simulink model "sampleModel193"  (R2021b)
settings: Solver=VariableStepAuto  StartTime=0.0  StopTime=10.0  RelTol=1e-3
undefined symbols (not defined in the file or in its folder): Newton, Raphson
libraries: simulink x7, slpidlib x2
settings Model: Creator=user  LastModifiedBy=user

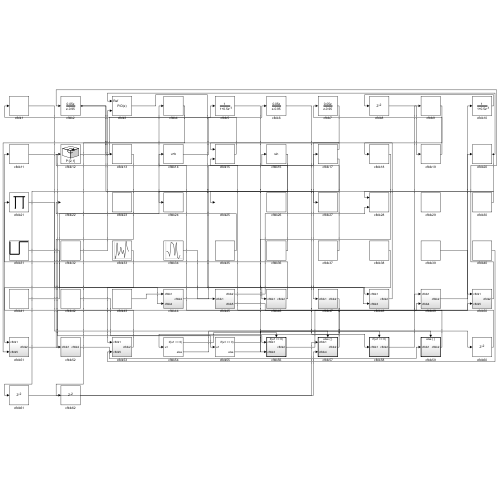
[thumbnail: Simulink's stored preview of the top-level diagram]
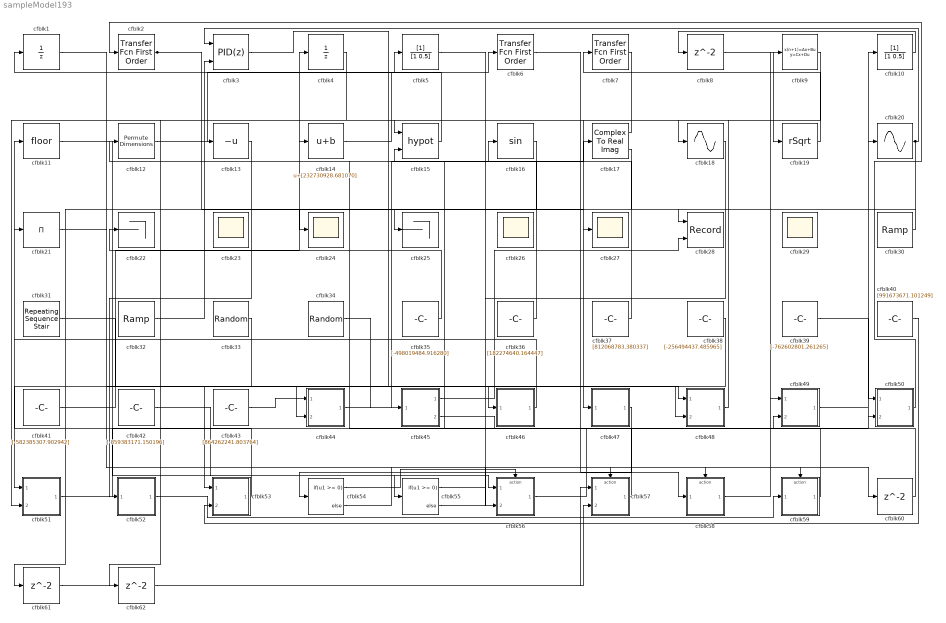
== system sampleModel193 ==
  cfblk1 : UnitDelay  HasFrameUpgradeWarning=on
  cfblk10 : DiscreteFilter  SampleTime=1
  cfblk11 : Rounding
  cfblk12 : PermuteDimensions
  cfblk13 : UnaryMinus
  cfblk14 : Bias  Bias=[232730928.681070]
  cfblk15 : Math  Operator=hypot  SaturateOnIntegerOverflow=on
  cfblk16 : Trigonometry
  cfblk17 : ComplexToRealImag
  cfblk18 : Sin  TimeSource=Use external signal  SampleTime=0
  cfblk19 : Sqrt  Operator=rSqrt  AlgorithmType=Newton-Raphson  SaturateOnIntegerOverflow=on
  cfblk2 : simulink/Discrete/Transfer Fcn First Order  PoleZ=0.95  ICPrevOutput=0.0  DoSatur=off
  cfblk20 : Sin  TimeSource=Use external signal  SampleTime=0
  cfblk21 : Product  Inputs=*
  cfblk22 : Terminator
  cfblk{23..24,26..27,29} (5 alike) : Scope
      cfblk23 settings: Floating=on
      cfblk26 settings: Floating=on
      cfblk29 settings: Floating=on
  cfblk25 : Terminator
  cfblk28 : Record  FileSettingsInternal="{\"entries\":[{\"content\":{\"excelSettings\":{\"content\":{},\"type\":\"Streamout.ExcelSettings\"}},\"type\":\"Streamout.FileSettingStorage\",\"uuid\":\"bc1bea57-7175-457e-a136-c385bfcfe488\"}],\"packageUris\":[\"http://schema.mathworks.com/mf0/streamout_blocks/R2020a\"],\"version\":\"1.0\"}"  Layout=[1 1]  SignalsInternal="{\"entries\":[{\"content\":{\"signals\":[{\"content\":{\"blockPath\":[\"sampleModel193/cfblk28\"],\"channel\":[],\"dimensions\":[1],\"domain\":\"sampleModel193/cfblk28\",\"lineColor\":\"#a2142f\",\"plots\":[1],\"port\":1,\"sid\":[\"\"],\"signalID\":7218,\"signalName\":\"cfblk30\"},\"type\":\"RecordBlkView.Signal\",\"uuid\":\"5325866a-24c1-4f14-81bb-e80c3d8cfcb1\"},{\"content\":{\"blockPath\":[\"sampleModel193/cfblk28\"],\"channel\":[],\"dimensions\":[1],\"domain\":\"sampleModel193/cfblk28\",\"lineColor\":\"#139fff\",\"plots\":[1],\"port\":2,\"sid\":[\"\"],\"signalID\":7222,\"signalName\":\"cfblk45:1\"},\"type\":\"RecordBlkView.Signal\",\"uuid\":\"43aee076-3444-4815-ba1f-177c12378f10\"}]},\"type\":\"RecordBlkView.InputSignals\",\"uuid\":\"ded13e2b-937f-46f2-b7aa-f57e1588ea0d\"}],\"packageUris\":[\"http://schema.mathworks.com/mf0/streamout_blocks/R2020a\"],\"version\":\"1.0\"}"  VisualizationBindings="{\"xyplotplugin\":{\"info\":[{\"series\":[{\"bindingParametersList\":[{\"parameter\":\"X-Axis\",\"signalID\":7218,\"signalName\":\"cfblk30\"},{\"parameter\":\"Y-Axis\",\"signalID\":7222,\"signalName\":\"cfblk45:1\"}],\"seriesID\":58629}],\"subplotID\":1}]}}"  CompatibilityTag=XY
  cfblk3 : slpidlib/PID Controller (2DOF)  Controller=PID  Form=Parallel  TimeDomain=Discrete-time  UseExternalTs=off  SampleTime=1  IntegratorMethod=Forward Euler  FilterMethod=Forward Euler  ControllerParametersSource=internal  P=1  I=1  D=0  UseFilter=on  N=100  b=1  c=1  TunerSelectOption=Transfer Function Based (PID Tuner App)  InitialConditionSource=internal  InitialConditionForIntegrator=0  InitialConditionForFilter=0  DifferentiatorICPrevScaledInput=0  ExternalReset=none  TrackingMode=off  Kt=1  LimitOutput=off  SatLimitsSource=internal  UpperSaturationLimit=inf  LowerSaturationLimit=-inf  LinearizeAsGain=off  AntiWindupMode=none  Kb=1  POutMin=[]  POutMax=[]  IOutMin=[]  IOutMax=[]  DOutMin=[]  DOutMax=[]  NOutMin=[]  NOutMax=[]  bOutMin=[]  bOutMax=[]  cOutMin=[]  cOutMax=[]  SumOutMin=[]  SumOutMax=[]  SaturationOutMin=[]  SaturationOutMax=[]  PParamMin=[]  PParamMax=[]  IParamMin=[]  IParamMax=[]  DParamMin=[]  DParamMax=[]  NParamMin=[]  NParamMax=[]  bParamMin=[]  bParamMax=[]  cParamMin=[]  cParamMax=[]  KbParamMin=[]  KbParamMax=[]  KtParamMin=[]  KtParamMax=[]  KbOutMin=[]  KbOutMax=[]  KtOutMin=[]  KtOutMax=[]  IntegratorOutMin=[]  IntegratorOutMax=[]  FilterOutMin=[]  FilterOutMax=[]  SumI1OutMin=[]  SumI1OutMax=[]  SumI2OutMin=[]  SumI2OutMax=[]  SumI3OutMin=[]  SumI3OutMax=[]  SumI4OutMin=[]  SumI4OutMax=[]  SumDOutMin=[]  SumDOutMax=[]  Sum1OutMin=[]  Sum1OutMax=[]  Sum2OutMin=[]  Sum2OutMax=[]  Sum3OutMin=[]  Sum3OutMax=[]  DifferentiatorOutMin=[]  DifferentiatorOutMax=[]  FilterDiffOutCoefMin=[]  FilterDiffOutCoefMax=[]  ReciprocalOutMin=[]  ReciprocalOutMax=[]  SumDenOutMin=[]  SumDenOutMax=[]  SumNumOutMin=[]  SumNumOutMax=[]  DivideOutMin=[]  DivideOutMax=[]  UdiffTsProdOutMin=[]  UdiffTsProdOutMax=[]  NTsProdOutMin=[]  NTsProdOutMax=[]  UintegralTsProdOutMin=[]  UintegralTsProdOutMax=[]  UngainTsProdOutMin=[]  UngainTsProdOutMax=[]  IntegratorContinuousStateAttributes=''  IntegratorStateMustResolveToSignalObject=off  IntegratorRTWStateStorageClass=Auto  FilterContinuousStateAttributes=''  FilterStateMustResolveToSignalObject=off  FilterRTWStateStorageClass=Auto  ParallelPVariant=InternalParameters  IdealPVariant=Disabled  IVariant=InternalParameters  DVariant=InternalParameters  bVariant=InternalParameters  cVariant=InternalParameters  IntegratorVariant=Discrete  SatVariant=Disabled  AWVariant=Passthrough  PCopyVariant=Disabled  TRVariant=Disabled  FdbkBlocksVariant=Forward  IdealPFdbkVariant=Disabled  SatFdbkVariant=Disabled  DerivativeFilterVariant=ForwardEulerFilter  NVariant=InternalParameters  NCopyVariant=Disabled  FilterICVariant=InternalICsFilter  IntegratorICVariant=InternalICs  ExternalResetVariant=Disabled  TRSumVariant=Passthrough  SumFdbkVariant=Disabled  SumVariant=Sum_PID  TsampFilterVariant=InternalTs  TsampNgainVariant=Passthrough  TsampIntegralVariant=Passthrough  ExternalSaturationOutDataTypeStr=Inherit: Same as second input
      settings: SourceProductBaseCode=SL
  cfblk30 : simulink/Sources/Ramp  slope=[-5810.697457]  start=[14.384632]  InitialOutput=[412696.799006]
  cfblk31 : simulink/Sources/Repeating Sequence Stair  OutValues=[-532873447.023768, -329477790.938633]  tsamp=-1  OutMin=[]  OutMax=[]  OutDataTypeStr=double  OutputDataTypeScalingMode=double  OutDataType=fixdt(0,8)  ConRadixGroup=Best Precision: Vector-wise  OutScaling=2^-12
  cfblk32 : simulink/Sources/Ramp  slope=[440.538023]  start=[2.948575]  InitialOutput=[-15658.111534]
  cfblk33 : UniformRandomNumber  Minimum=[-942132288.166952]  Maximum=[1760766452.681617]  Seed=[86964386.000000]  SampleTime=0.1
  cfblk34 : RandomNumber  Mean=[43865.707237]  Variance=[65444.635651]  Seed=[951810309.000000]  SampleTime=0.1
  cfblk35 : Constant  Value=[-498019484.916280]  SampleTime=1
  cfblk36 : Constant  Value=[182274640.164447]  SampleTime=1
  cfblk37 : Constant  Value=[812068783.380337]  SampleTime=1
  cfblk38 : Constant  Value=[-256494437.485965]  SampleTime=1
  cfblk39 : Constant  Value=[-762602801.261265]  SampleTime=1
  cfblk4 : UnitDelay  HasFrameUpgradeWarning=on
  cfblk40 : Constant  Value=[991673671.101249]  SampleTime=1
  cfblk41 : Constant  Value=[-582385307.902942]  SampleTime=1
  cfblk42 : Constant  Value=[-859383171.150196]  SampleTime=1
  cfblk43 : Constant  Value=[864262241.803764]  SampleTime=1
  cfblk44 : Subsystem
  cfblk45 : Subsystem
  cfblk46 : Subsystem
  cfblk47 : Subsystem
  cfblk48 : Subsystem
  cfblk49 : Subsystem
  cfblk5 : DiscreteFilter  SampleTime=1
  cfblk50 : Subsystem
  cfblk51 : Subsystem
  cfblk52 : Subsystem
  cfblk53 : Subsystem
  cfblk54 : If  IfExpression=u1 >= 0  SampleTime=1
  cfblk55 : If  IfExpression=u1 >= 0  SampleTime=1
  cfblk56 : Subsystem  TreatAsAtomicUnit=on
  cfblk57 : Subsystem  TreatAsAtomicUnit=on
  cfblk58 : Subsystem  TreatAsAtomicUnit=on
  cfblk59 : Subsystem  TreatAsAtomicUnit=on
  cfblk6 : simulink/Discrete/Transfer Fcn First Order  PoleZ=0.95  ICPrevOutput=0.0  DoSatur=off
  cfblk{8,60..62} (4 alike) : Delay  SampleTime=1
  cfblk7 : simulink/Discrete/Transfer Fcn First Order  PoleZ=0.95  ICPrevOutput=0.0  DoSatur=off
  cfblk9 : DiscreteStateSpace
  wires:
  cfblk34/1 -> cfblk45/1(cfblk1)
  cfblk41/1 -> cfblk4/1
  cfblk17/1 -> cfblk15/1
  cfblk51/1(cfblk2) -> cfblk10/1
  cfblk19/1 -> cfblk7/1
  cfblk33/1 -> cfblk51/1(cfblk1)
  cfblk52/1(cfblk2) -> cfblk59/1(cfblk1)
  cfblk3/1 -> cfblk46/1(cfblk1)
  cfblk38/1 -> cfblk53/1(cfblk1)
  cfblk15/1 -> cfblk1/1
  cfblk47/1(cfblk2) -> cfblk54/1
  cfblk49/1(cfblk2) -> cfblk20/1
  cfblk36/1 -> cfblk16/1
  cfblk43/1 -> cfblk44/1(cfblk1)
  cfblk6/1 -> cfblk58/1(cfblk1)
  cfblk59/1(cfblk2) -> cfblk15/2
  cfblk11/1 -> cfblk56/1(cfblk1)
  cfblk31/1 -> cfblk44/2(cfblk4)
  cfblk35/1 -> cfblk22/1
  cfblk18/1 -> cfblk56/2(cfblk3)
  cfblk16/1 -> cfblk24/1
  cfblk37/1 -> cfblk12/1
  cfblk8/1 -> cfblk19/1
  cfblk53/1(cfblk2) -> cfblk11/1
  cfblk17/2 -> cfblk25/1
  cfblk14/1 -> cfblk6/1
  cfblk40/1 -> cfblk53/2(cfblk5)
  cfblk42/1 -> cfblk55/1
  cfblk4/1 -> cfblk51/2(cfblk5)
  cfblk20/1 -> cfblk3/1, cfblk61/1
  cfblk10/1 -> cfblk8/1
  cfblk58/1(cfblk2) -> cfblk9/1
  cfblk12/1 -> cfblk5/1
  cfblk46/1(cfblk2) -> cfblk21/1
  cfblk7/1 -> cfblk47/1(cfblk1)
  cfblk50/1(cfblk2) -> cfblk2/1
  cfblk5/1 -> cfblk48/1(cfblk1)
  cfblk32/1 -> cfblk3/2
  cfblk39/1 -> cfblk50/1(cfblk1)
  cfblk48/1(cfblk2) -> cfblk18/1
  cfblk44/1(cfblk2) -> cfblk17/1
  cfblk30/1 -> cfblk28/1
  cfblk1/1 -> cfblk48/2(cfblk3)
  cfblk56/1(cfblk2) -> cfblk49/2(cfblk4)
  cfblk2/1 -> cfblk13/1, cfblk27/1
  cfblk57/1(cfblk2) -> cfblk14/1
  cfblk13/1 -> cfblk52/1(cfblk1)
  cfblk45/1(cfblk2) -> cfblk28/2
  cfblk45/2(cfblk5) -> cfblk50/2(cfblk5)
  cfblk54/1 -> cfblk56/Action
  cfblk54/2 -> cfblk57/Action
  cfblk55/1 -> cfblk58/Action
  cfblk55/2 -> cfblk59/Action
  cfblk21/1 -> cfblk60/1
  cfblk60/1 -> cfblk49/1(cfblk1)
  cfblk61/1 -> cfblk57/2(cfblk4)
  cfblk9/1 -> cfblk62/1
  cfblk62/1 -> cfblk57/1(cfblk1)

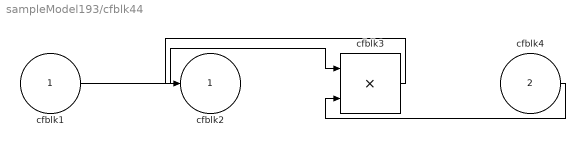
== system sampleModel193/cfblk44 ==
  cfblk1 : Inport
  cfblk4 : Inport  Port=2
  cfblk3 : Product  Inputs=**
  cfblk2 : Outport
  wires:
  cfblk1/1 -> cfblk3/1
  cfblk4/1 -> cfblk3/2
  cfblk3/1 -> cfblk2/1

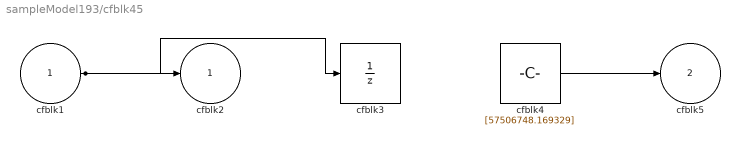
== system sampleModel193/cfblk45 ==
  cfblk1 : Inport
  cfblk3 : UnitDelay  HasFrameUpgradeWarning=on
  cfblk4 : Constant  Value=[57506748.169329]  SampleTime=1
  cfblk2 : Outport
  cfblk5 : Outport  Port=2
  wires:
  cfblk1/1 -> cfblk2/1, cfblk3/1
  cfblk4/1 -> cfblk5/1

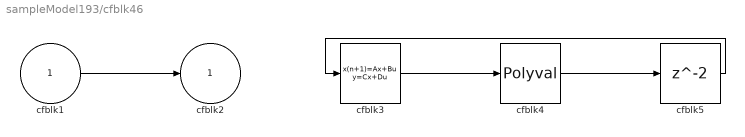
== system sampleModel193/cfblk46 ==
  cfblk1 : Inport
  cfblk3 : DiscreteStateSpace
  cfblk4 : Polyval  Coefs=[ +2.081618890e-019, -1.441693666e-014, +4.719686976e-010, -8.536869453e-006, +1.621573104e-001, -8.087801117e+001 ]
  cfblk5 : Delay  SampleTime=1
  cfblk2 : Outport
  wires:
  cfblk1/1 -> cfblk2/1
  cfblk3/1 -> cfblk4/1
  cfblk4/1 -> cfblk5/1
  cfblk5/1 -> cfblk3/1

== system sampleModel193/cfblk47 ==
  cfblk1 : Inport
  cfblk3 : Constant  Value=[-884953011.251367]  SampleTime=1
  cfblk2 : Outport
  wires:
  cfblk3/1 -> cfblk2/1

== system sampleModel193/cfblk48 ==
  cfblk1 : Inport
  cfblk3 : Inport  Port=2
  cfblk2 : Outport
  wires:
  cfblk3/1 -> cfblk2/1

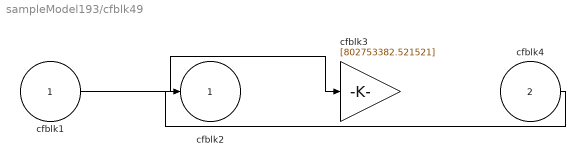
== system sampleModel193/cfblk49 ==
  cfblk1 : Inport
  cfblk4 : Inport  Port=2
  cfblk3 : Gain  Gain=[802753382.521521]
  cfblk2 : Outport
  wires:
  cfblk1/1 -> cfblk3/1
  cfblk4/1 -> cfblk2/1

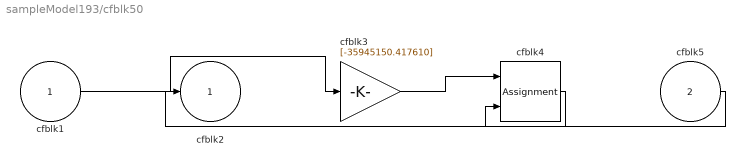
== system sampleModel193/cfblk50 ==
  cfblk1 : Inport
  cfblk5 : Inport  Port=2
  cfblk3 : Gain  Gain=[-35945150.417610]
  cfblk4 : Assignment  DiagnosticForDimensions=Warning  IndexOptions=Index vector (dialog)  Indices=1  OutputSizes=1
  cfblk2 : Outport
  wires:
  cfblk3/1 -> cfblk4/1
  cfblk1/1 -> cfblk3/1
  cfblk4/1 -> cfblk2/1
  cfblk5/1 -> cfblk4/2

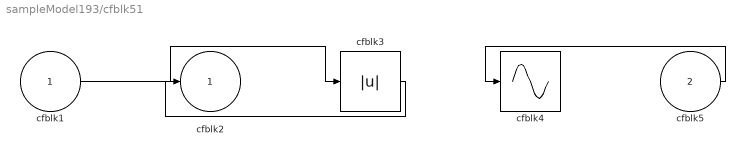
== system sampleModel193/cfblk51 ==
  cfblk1 : Inport
  cfblk5 : Inport  Port=2
  cfblk3 : Abs
  cfblk4 : Sin  TimeSource=Use external signal  SampleTime=0
  cfblk2 : Outport
  wires:
  cfblk5/1 -> cfblk4/1
  cfblk1/1 -> cfblk3/1
  cfblk3/1 -> cfblk2/1

== system sampleModel193/cfblk52 ==
  cfblk1 : Inport
  cfblk3 : slpidlib/PID Controller  Controller=PID  Form=Parallel  TimeDomain=Discrete-time  UseExternalTs=off  SampleTime=1  IntegratorMethod=Forward Euler  FilterMethod=Forward Euler  ControllerParametersSource=internal  P=1  I=1  D=0  UseFilter=on  N=100  TunerSelectOption=Transfer Function Based (PID Tuner App)  InitialConditionSource=internal  InitialConditionForIntegrator=0  InitialConditionForFilter=0  DifferentiatorICPrevScaledInput=0  ExternalReset=none  TrackingMode=off  Kt=1  LimitOutput=off  SatLimitsSource=internal  UpperSaturationLimit=inf  LowerSaturationLimit=-inf  LinearizeAsGain=off  AntiWindupMode=none  Kb=1  POutMin=[]  POutMax=[]  IOutMin=[]  IOutMax=[]  DOutMin=[]  DOutMax=[]  NOutMin=[]  NOutMax=[]  SumOutMin=[]  SumOutMax=[]  SaturationOutMin=[]  SaturationOutMax=[]  PParamMin=[]  PParamMax=[]  IParamMin=[]  IParamMax=[]  DParamMin=[]  DParamMax=[]  NParamMin=[]  NParamMax=[]  KbParamMin=[]  KbParamMax=[]  KtParamMin=[]  KtParamMax=[]  KbOutMin=[]  KbOutMax=[]  KtOutMin=[]  KtOutMax=[]  IntegratorOutMin=[]  IntegratorOutMax=[]  FilterOutMin=[]  FilterOutMax=[]  SumI1OutMin=[]  SumI1OutMax=[]  SumI2OutMin=[]  SumI2OutMax=[]  SumI3OutMin=[]  SumI3OutMax=[]  SumI4OutMin=[]  SumI4OutMax=[]  SumDOutMin=[]  SumDOutMax=[]  DifferentiatorOutMin=[]  DifferentiatorOutMax=[]  FilterDiffOutCoefMin=[]  FilterDiffOutCoefMax=[]  ReciprocalOutMin=[]  ReciprocalOutMax=[]  SumDenOutMin=[]  SumDenOutMax=[]  SumNumOutMin=[]  SumNumOutMax=[]  DivideOutMin=[]  DivideOutMax=[]  UdiffTsProdOutMin=[]  UdiffTsProdOutMax=[]  NTsProdOutMin=[]  NTsProdOutMax=[]  UintegralTsProdOutMin=[]  UintegralTsProdOutMax=[]  UngainTsProdOutMin=[]  UngainTsProdOutMax=[]  IntegratorContinuousStateAttributes=''  IntegratorStateMustResolveToSignalObject=off  IntegratorRTWStateStorageClass=Auto  FilterContinuousStateAttributes=''  FilterStateMustResolveToSignalObject=off  FilterRTWStateStorageClass=Auto  ParallelPVariant=InternalParameters  IdealPVariant=Disabled  IVariant=InternalParameters  DVariant=InternalParameters  IntegratorVariant=Discrete  SatVariant=Disabled  AWVariant=Passthrough  PCopyVariant=Disabled  TRVariant=Disabled  FdbkBlocksVariant=Forward  IdealPFdbkVariant=Disabled  SatFdbkVariant=Disabled  DerivativeFilterVariant=ForwardEulerFilter  NVariant=InternalParameters  NCopyVariant=Disabled  FilterICVariant=InternalICsFilter  IntegratorICVariant=InternalICs  ExternalResetVariant=Disabled  TRSumVariant=Passthrough  SumFdbkVariant=Disabled  SumVariant=Sum_PID  TsampFilterVariant=InternalTs  TsampNgainVariant=Passthrough  TsampIntegralVariant=Passthrough  ExternalSaturationOutDataTypeStr=Inherit: Same as second input
  cfblk2 : Outport
  wires:
  cfblk1/1 -> cfblk3/1
  cfblk3/1 -> cfblk2/1

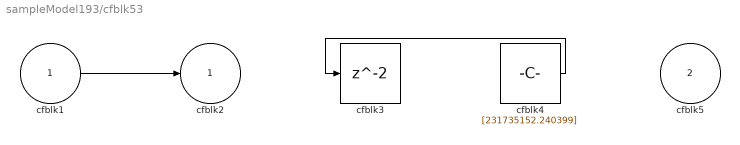
== system sampleModel193/cfblk53 ==
  cfblk1 : Inport
  cfblk5 : Inport  Port=2
  cfblk3 : Delay  SampleTime=1
  cfblk4 : Constant  Value=[231735152.240399]  SampleTime=1
  cfblk2 : Outport
  wires:
  cfblk1/1 -> cfblk2/1
  cfblk4/1 -> cfblk3/1

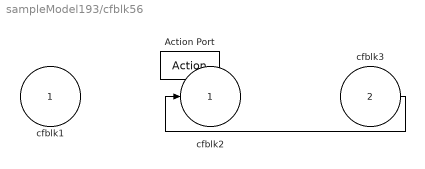
== system sampleModel193/cfblk56 ==
  cfblk1 : Inport
  cfblk3 : Inport  Port=2
  Action Port : ActionPort  ActionPortLabel=if(u1 >= 0)
  cfblk2 : Outport
  wires:
  cfblk3/1 -> cfblk2/1

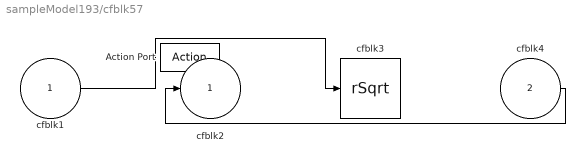
== system sampleModel193/cfblk57 ==
  cfblk1 : Inport
  cfblk4 : Inport  Port=2
  Action Port : ActionPort  ActionPortLabel=else
  cfblk3 : Sqrt  Operator=rSqrt  AlgorithmType=Newton-Raphson  SaturateOnIntegerOverflow=on
  cfblk2 : Outport
  wires:
  cfblk4/1 -> cfblk2/1
  cfblk1/1 -> cfblk3/1

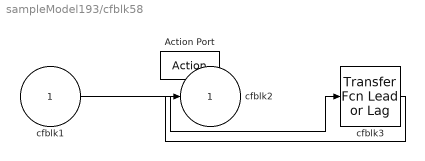
== system sampleModel193/cfblk58 ==
  cfblk1 : Inport
  Action Port : ActionPort  ActionPortLabel=if(u1 >= 0)
  cfblk3 : simulink/Discrete/Transfer Fcn Lead or Lag  PoleZ=0.95  ZeroZ=0.75  ICPrevOutput=0.0  ICPrevInput=0.0  DoSatur=off
      settings: SourceProductBaseCode=SL
  cfblk2 : Outport
  wires:
  cfblk1/1 -> cfblk3/1
  cfblk3/1 -> cfblk2/1

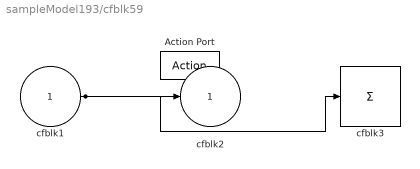
== system sampleModel193/cfblk59 ==
  cfblk1 : Inport
  Action Port : ActionPort  ActionPortLabel=else
  cfblk3 : Sum  Inputs=+
  cfblk2 : Outport
  wires:
  cfblk1/1 -> cfblk2/1, cfblk3/1
